simulink model "path2"  (R2023a)
settings: Solver=VariableStepAuto  StartTime=0.0  StopTime=10.0  RelTol=1e-3
undefined symbols (not defined in the file or in its folder): DiscIntNeverNeededParam
settings Model: Creator=jiaweichen  LastModifiedBy=jiaweichen
settings OptimizationCC: ReuseModelBlockBuffer=off

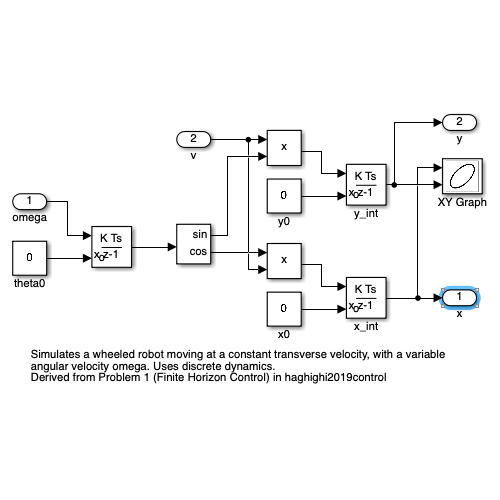
[thumbnail: Simulink's stored preview of the top-level diagram]
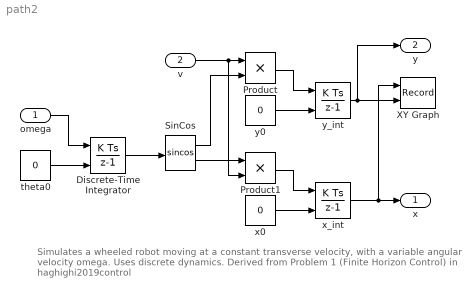
== system path2 ==
  note: Simulates a wheeled robot moving at a constant transverse velocity, with a variable angular velocity omega. Uses discrete dynamics.
      | Derived from Problem 1 (Finite Horizon Control) in haghighi2019control
  omega : Inport
  v : Inport  Port=2
  Discrete-Time Integrator : DiscreteIntegrator  InitialConditionSource=external  SampleTime=0.1  ICPrevOutput=DiscIntNeverNeededParam  ICPrevScaledInput=DiscIntNeverNeededParam
  Product : Product
  Product1 : Product
  SinCos : Trigonometry  Operator=sincos
  XY Graph : Record  FileSettingsInternal="{\"entries\":[{\"content\":{\"excelSettings\":{\"content\":{},\"type\":\"Streamout.ExcelSettings\"}},\"type\":\"Streamout.FileSettingStorage\",\"uuid\":\"6e87e3c9-b38b-4ac3-b2fe-6a34d160bf9e\"}],\"packageUris\":[\"http://schema.mathworks.com/mf0/streamout_blocks/R2020a\"],\"version\":\"1.0\"}"  Layout=[1 1]  SignalsInternal="{\"entries\":[{\"content\":{\"signals\":[{\"content\":{\"blockPath\":[\"path2/XY Graph\"],\"dimensions\":[1],\"domain\":\"path2/XY Graph\",\"lineColor\":\"#a2142f\",\"plots\":[1],\"port\":1,\"signalID\":200,\"signalName\":\"x\"},\"type\":\"RecordBlkView.Signal\",\"uuid\":\"277cd461-cebd-4884-8d3c-3cc32acac323\"},{\"content\":{\"blockPath\":[\"path2/XY Graph\"],\"dimensions\":[1],\"domain\":\"path2/XY Graph\",\"lineColor\":\"#139fff\",\"plots\":[1],\"port\":2,\"signalID\":203,\"signalName\":\"y\"},\"type\":\"RecordBlkView.Signal\",\"uuid\":\"aac1630d-fd1f-402f-b236-60c3985104a6\"}]},\"type\":\"RecordBlkView.InputSignals\",\"uuid\":\"4e404feb-34e5-45ab-993e-dbcf9c8c8622\"}],\"packageUris\":[\"http://schema.mathworks.com/mf0/streamout_blocks/R2020a\"],\"version\":\"1.0\"}"  VisualizationBindings="{\"xyplotplugin\":{\"info\":[{\"series\":[{\"bindingParametersList\":[{\"parameter\":\"X-Axis\",\"signalID\":200,\"signalName\":\"x\"},{\"parameter\":\"Y-Axis\",\"signalID\":203,\"signalName\":\"y\"}],\"seriesID\":63123}],\"subplotID\":1}]}}"  CompatibilityTag=XY
  theta0 : Constant  Value=0
  x0 : Constant  Value=0
  x_int : DiscreteIntegrator  InitialConditionSource=external  SampleTime=0.1  ICPrevOutput=DiscIntNeverNeededParam  ICPrevScaledInput=DiscIntNeverNeededParam
  y0 : Constant  Value=0
  y_int : DiscreteIntegrator  InitialConditionSource=external  SampleTime=0.1  ICPrevOutput=DiscIntNeverNeededParam  ICPrevScaledInput=DiscIntNeverNeededParam
  x : Outport
  y : Outport  Port=2
  wires:
  x_int/1 -> x/1, XY Graph/1
  Discrete-Time Integrator/1 -> SinCos/1
  x0/1 -> x_int/2
  Product/1 -> y_int/1
  y0/1 -> y_int/2
  y_int/1 -> y/1, XY Graph/2
  SinCos/2 -> Product1/1
  SinCos/1 -> Product/2
  v/1 -> Product/1, Product1/2
  Product1/1 -> x_int/1
  theta0/1 -> Discrete-Time Integrator/2
  omega/1 -> Discrete-Time Integrator/1
